simulink model "AllCheckoutsSim"  (R2020a)
settings: Solver=VariableStepAuto  StartTime=0.0  StopTime=2000000  RelTol=1e-3
InitFcn:
  | SimulationParameters
values from neighbouring files (symbols this model uses):
  NumExpressCheckouts = 2    [Sandbox.m]    (also in SimWrapper.m = NumExpressCheckoutsVec(i); SimulationParameters.m = Inputs(2))
  NumExpressCheckoutsHelper = NumExpressCheckouts    (= 2)    [Sandbox.m]    (also in SimulationParameters.m = NumExpressCheckouts)
  NumRegularCheckouts = 7    [Sandbox.m]    (also in SimWrapper.m = NumRegularCheckoutsVec(i); SimulationParameters.m = Inputs(1))
  NumRegularCheckoutsHelper = NumRegularCheckouts    (= 7)    [Sandbox.m]    (also in SimulationParameters.m = NumRegularCheckouts)
  NumSelfCheckouts = 2    [Sandbox.m]    (also in SimWrapper.m = NumSelfCheckoutsVec(i); SimulationParameters.m = Inputs(3))
  NumSelfCheckoutsHelper = NumSelfCheckouts    (= 2)    [Sandbox.m]    (also in SimulationParameters.m = NumSelfCheckouts)
  QueueCapacity = 7    [Sandbox.m]    (also in SimWrapper.m = QueueCapacityVec(i); SimulationParameters.m = Inputs(4))
undefined symbols (not defined in the file or in its folder): m, n
libraries: dspindex x3, dspstat3 x3
settings Model: Creator=jggam  LastModifiedBy=jggam

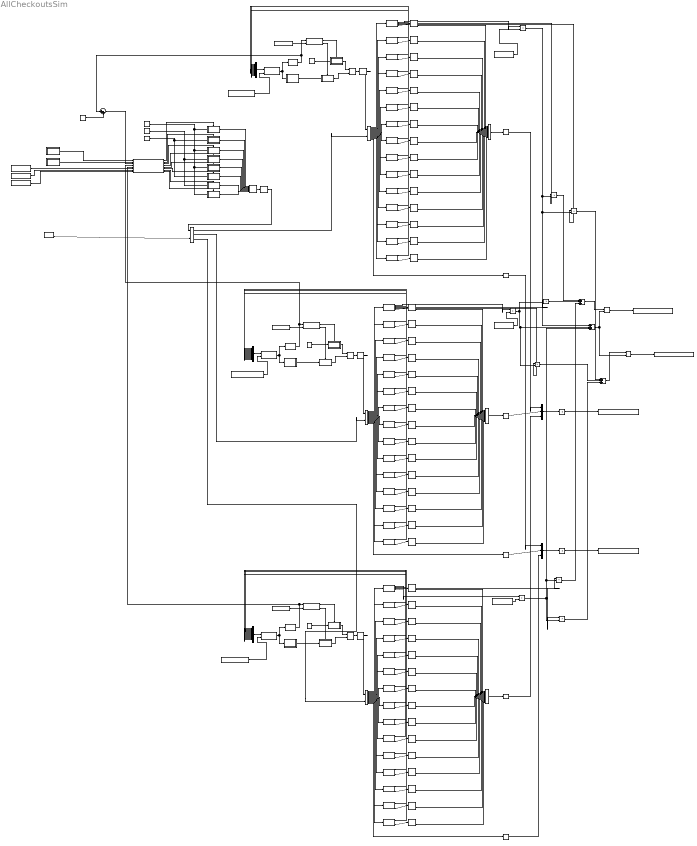
== system AllCheckoutsSim ==
  note: u1 = BelowItemsThresh
      | u2 = SelfCheckoutEligibile
      | u3 = Min Length of Regular
      | u4 = Min Length of Express
      | u5 = Min Length of Self
      | u6 = NumRegularCheckouts
      | u7 = NumExpressCheckouts
      | u8 = NumSelfCheckouts
  note: Hello! Welcome to the simulation of checkouts at a grocery store.
      | In order to change the queue capacities, number of each type of checkouts, item limit, and time of day,
      | 	change the variables at the top of the SimulationParameters.m file in MATLAB.
      |
      | You can have between 0 and 15 checkouts of each type, but make sure to always use at least 1 regular checkout.
      | Generally, your wait times will get much shorter is you use more than 9 or 10 total checkouts.
      |
      | You don't need to run the file, just change the variables and save the file.
      | After saving the SimulationParameters.m file, you can open the Data Inspector at the top of Simulink,
      | 	then Run the simulation.
      |
      | In the Data Inspector, there are a few signals that you can view. If you sort the signals by Name, they'll be grouped by type.
      | 	A. Average wait times for each type of checkout and overall.
      | 	B. Number of customers serviced by each type of checkout and overall.
      | 	C. Number of customers lost by each type of checkout and overall. I would only use the overall value here.
      | 	D. Average number of customers for each type of checkout and overall.
      | 	E. Current number of customers over time for each type of checkout and overall.
      | 	F. Total customers arrived to the simulation.
  A. Overall Average Wait Time : Product  Inputs=*/
  Add : Sum  Inputs=+++
  Add1 : Sum  Inputs=+++
  Add2 : Sum  Inputs=+++
  Aggregate all queue lengths : Concatenate  NumInputs=15
  Aggregate all queue lengths1 : Concatenate  NumInputs=15
  Aggregate all queue lengths2 : Concatenate  NumInputs=15
  B. Express Serviced Customers : EntityTerminator  InputPortMessageModes=m  NumberEntitiesArrived=on
      settings: OutputPortMap=o0
  B. Regular Serviced Customers : EntityTerminator  InputPortMessageModes=m  NumberEntitiesArrived=on
      settings: OutputPortMap=o0
  B. Self Serviced Customers : EntityTerminator  InputPortMessageModes=m  NumberEntitiesArrived=on
      settings: OutputPortMap=o0
  B. Total Serviced Customers : Sum  Inputs=+
  C. Express Lost Customers : EntityTerminator  InputPortMessageModes=m  NumberEntitiesArrived=on
      settings: OutputPortMap=o0
  C. Regular Lost Customers : EntityTerminator  InputPortMessageModes=m  NumberEntitiesArrived=on
      settings: OutputPortMap=o0
  C. Self Lost Customers : EntityTerminator  InputPortMessageModes=m  NumberEntitiesArrived=on
      settings: OutputPortMap=o0
  C. Total Lost Customers : Sum  Inputs=+
  Concatenate : Concatenate  NumInputs=3
  Concatenate1 : Concatenate  NumInputs=3
  Constant : Constant  Value=QueueCapacity
  Constant1 : Constant  Value=QueueCapacity
  Constant10 : Constant  Value=[1:NumSelfCheckoutsHelper]
  Constant13 : Constant  Value=[1:NumExpressCheckoutsHelper]
  Constant2 : Constant  Value=QueueCapacity
  Constant3 : Constant  Value=NumRegularCheckouts
  Constant4 : Constant  Value=NumRegularCheckouts
  Constant5 : Constant  Value=NumExpressCheckouts
  Constant6 : Constant  Value=NumExpressCheckouts
  Constant7 : Constant  Value=NumSelfCheckouts
  Constant8 : Constant  Value=[1:NumRegularCheckoutsHelper]
  Constant9 : Constant  Value=NumSelfCheckouts
  Customer Arrivals : EntityGenerator  OutputPortMessageModes=n,m  TimeSource=MATLAB action  Period=0.5  IntergenerationTimeAction=dt = arrivalTime(RandArrivalTimesDist);  GenerateEntityAtSimulationStart=off  GenerateAction=|  ExitAction=|  AttributeName=NumberOfItems|BelowItemThresh|SelfCheckoutEligible  AttributeInitialValue=1|false|false  NumberEntitiesDeparted=on  EntityType=Structured  EntityTypeName=Entity
      GenerateAction=|
      | entity.NumberOfItems = numberOfItems(RandItemsDist);
      | if entity.NumberOfItems <= SelfAndExpressMaxItems
      |     entity.BelowItemThresh = true;
      | end
      | if rand() < AmountSelfCheckoutEligible
      |     entity.SelfCheckoutEligible = true;
      | end
      ExitAction=|
      | observeBelowItemThresh(entity.BelowItemThresh);
      | observeEligibility(entity.SelfCheckoutEligible);
      settings: OutputPortMap=o0,o3
  D. Overall Average # of Customers Waiting : Product  Inputs=*/
  Determine which queue to send to : Merge
  Determine which queue to send to1 : Merge
  Determine which queue to send to2 : Merge
  Entity Input Switch : EntityInputSwitch  InputPortMessageModes=m,m,m,m,m,m,m,m,m,m,m,m,m,m,m  OutputPortMessageModes=m  NumberInputPorts=15
      settings: InputPortMap=u1,u2,u3,u4,u5,u6,u7,u8,u9,u10,u11,u12,u13,u14,u15
  Entity Input Switch1 : EntityInputSwitch  InputPortMessageModes=m,m,m,m,m,m,m,m,m,m,m,m,m,m,m  OutputPortMessageModes=m  NumberInputPorts=15
      settings: InputPortMap=u1,u2,u3,u4,u5,u6,u7,u8,u9,u10,u11,u12,u13,u14,u15
  Entity Input Switch2 : EntityInputSwitch  InputPortMessageModes=m,m,m,m,m,m,m,m,m,m,m,m,m,m,m  OutputPortMessageModes=m  NumberInputPorts=15
      settings: InputPortMap=u1,u2,u3,u4,u5,u6,u7,u8,u9,u10,u11,u12,u13,u14,u15
  Entity Output Switch : EntityOutputSwitch  InputPortMessageModes=m,m  OutputPortMessageModes=m,m,m,m,m,m,m,m,m,m,m,m,m,m,m,m  NumberOutputPorts=16  SwitchingCriterion=From control port  SwitchAttributeName=Attribute1
      settings: InputPortMap=u0,u1  OutputPortMap=o0,o1,o2,o3,o4,o5,o6,o7,o8,o9,o10,o11,o12,o13,o14,o15
  Entity Output Switch1 : EntityOutputSwitch  InputPortMessageModes=m,m  OutputPortMessageModes=m,m,m,m,m,m,m,m,m,m,m,m,m,m,m,m  NumberOutputPorts=16  SwitchingCriterion=From control port  SwitchAttributeName=Attribute1
      settings: InputPortMap=u0,u1  OutputPortMap=o0,o1,o2,o3,o4,o5,o6,o7,o8,o9,o10,o11,o12,o13,o14,o15
  Entity Output Switch2 : EntityOutputSwitch  InputPortMessageModes=m,m  OutputPortMessageModes=m,m,m,m,m,m,m,m,m,m,m,m,m,m,m,m  NumberOutputPorts=16  SwitchingCriterion=From control port  SwitchAttributeName=Attribute1
      settings: InputPortMap=u0,u1  OutputPortMap=o0,o1,o2,o3,o4,o5,o6,o7,o8,o9,o10,o11,o12,o13,o14,o15
  Entity Output Switch3 : EntityOutputSwitch  InputPortMessageModes=m,m  OutputPortMessageModes=m,m,m  NumberOutputPorts=3  SwitchingCriterion=From control port  SwitchAttributeName=Attribute1
      settings: InputPortMap=u0,u1  OutputPortMap=o0,o1,o2
  Express Checkout : Constant  Value=2
  Express Queue1 : Queue  InputPortMessageModes=m  OutputPortMessageModes=n,n,n,n,m  Capacity=QueueCapacity  NumberEntitiesDeparted=on  NumberEntitiesInBlock=on  AverageWait=on  AverageQueueLength=on
      settings: OutputPortMap=o0,o1,o2,o3,o5
  Express Queue{2..15} (14 alike) : Queue  InputPortMessageModes=m  OutputPortMessageModes=n,n,n,m  Capacity=QueueCapacity  NumberEntitiesInBlock=on  AverageWait=on  AverageQueueLength=on
      settings: OutputPortMap=o1,o2,o3,o5
  Express Server{1..15} (15 alike) : EntityServer  InputPortMessageModes=m  OutputPortMessageModes=n,m  Capacity=1  ServiceTimeSource=MATLAB action  ServiceTimeValue=1.75  ServiceTimeAction=dt = expressServiceTime(RandExpressServiceTimesDist);  AverageWait=on
      settings: OutputPortMap=o4,o9
  Go to Regular : Subsystem  TreatAsAtomicUnit=on
  If : If  NumInputs=2  IfExpression=u1 == u2  ZeroCross=off
  If for self checkouts : If  NumInputs=8  IfExpression=u7 == 0 & u8 == 0  ElseIfExpressions=u7 == 0 & u1 & u2 & u5 <= u3, u7 == 0, u8 == 0 & u1 & u4 <= u3, u8 == 0, u1 & u2 & u5 <= u3 & u5 <= u4, u1 & u4 <= u3  ZeroCross=off
  "If shortest queue is full, remove this customer" : Subsystem  TreatAsAtomicUnit=on
  "If shortest queue is full, remove this customer1" : Subsystem  TreatAsAtomicUnit=on
  "If shortest queue is full, remove this customer2" : Subsystem  TreatAsAtomicUnit=on
  "If there are no express or self, send to regular" : Subsystem  TreatAsAtomicUnit=on
  "If there are no express, and we're under items limit, and we're eligible for self, and the regular queues aren't shorter than self, go to self" : Subsystem  TreatAsAtomicUnit=on
  "If there are no express, go to regular" : Subsystem  TreatAsAtomicUnit=on
  "If there are no self, and we're under the items limit, and the regular queues aren't shorter than express, go to express" : Subsystem  TreatAsAtomicUnit=on
  "If there are no self, go to regular" : Subsystem  TreatAsAtomicUnit=on
  "If we're under the items limit and eligible for self and the regular and express queues aren't shorter than self, go to self" : Subsystem  TreatAsAtomicUnit=on
  "If we're under the items limit and the regular queue isn't shorter than express, go to express" : Subsystem  TreatAsAtomicUnit=on
  If1 : If  NumInputs=2  IfExpression=u1 == u2  ZeroCross=off
  If2 : If  NumInputs=2  IfExpression=u1 == u2  ZeroCross=off
  Index of exit queue : Constant  Value=16
  Index of exit queue1 : Constant  Value=16
  Index of exit queue2 : Constant  Value=16
  Only use open registers : dspindex/Variable Selector  NumInputs=1  rowsOrCols=Rows  IdxMode=Variable  Elements=16  ZerOneIdxMode=One-based  errmode=Clip Index  FillMode=off  FillValues=0
  Only use open registers1 : dspindex/Variable Selector  NumInputs=1  rowsOrCols=Rows  IdxMode=Variable  Elements=[16]  ZerOneIdxMode=One-based  errmode=Clip Index  FillMode=on  FillValues=0
  Only use open registers2 : dspindex/Variable Selector  NumInputs=1  rowsOrCols=Rows  IdxMode=Variable  Elements=[16]  ZerOneIdxMode=One-based  errmode=Clip Index  FillMode=on  FillValues=0
  "Otherwise, send customer to random shortest queue" : Subsystem  TreatAsAtomicUnit=on
  "Otherwise, send customer to random shortest queue1" : Subsystem  TreatAsAtomicUnit=on
  "Otherwise, send customer to random shortest queue2" : Subsystem  TreatAsAtomicUnit=on
  Product{,1..8} (9 alike) : Product
  Random index of shortest queue length : MATLAB Function  TreatAsAtomicUnit=on
  Random index of shortest queue length1 : MATLAB Function  TreatAsAtomicUnit=on
  Random index of shortest queue length2 : MATLAB Function  TreatAsAtomicUnit=on
  Regular Checkout : Constant
  Regular Checkout Offset : Constant  Value=0
  Regular Queue1 : Queue  InputPortMessageModes=m  OutputPortMessageModes=n,n,n,n,m  Capacity=QueueCapacity  NumberEntitiesDeparted=on  NumberEntitiesInBlock=on  AverageWait=on  AverageQueueLength=on
      settings: OutputPortMap=o0,o1,o2,o3,o5
  Regular Queue{2..15} (14 alike) : Queue  InputPortMessageModes=m  OutputPortMessageModes=n,n,n,m  Capacity=QueueCapacity  NumberEntitiesInBlock=on  AverageWait=on  AverageQueueLength=on
      settings: OutputPortMap=o1,o2,o3,o5
  Regular Server1 : EntityServer  InputPortMessageModes=m  OutputPortMessageModes=n,m  Capacity=1  ServiceTimeSource=MATLAB action  ServiceTimeValue=1.75  ServiceTimeAction=|  AverageWait=on
      | if entity.BelowItemThresh
      |     dt = expressServiceTime(RandExpressServiceTimesDist);
      | else
      |     dt = regularServiceTime(RandRegularServiceTimesDist);
      settings: OutputPortMap=o4,o9
  Regular Server10 : EntityServer  InputPortMessageModes=m  OutputPortMessageModes=n,m  Capacity=1  ServiceTimeSource=MATLAB action  ServiceTimeValue=1.75  ServiceTimeAction=|  AverageWait=on
      | if entity.BelowItemThresh
      |     dt = expressServiceTime(RandExpressServiceTimesDist);
      | else
      |     dt = regularServiceTime(RandRegularServiceTimesDist);
      settings: OutputPortMap=o4,o9
  Regular Server11 : EntityServer  InputPortMessageModes=m  OutputPortMessageModes=n,m  Capacity=1  ServiceTimeSource=MATLAB action  ServiceTimeValue=1.75  ServiceTimeAction=|  AverageWait=on
      | if entity.BelowItemThresh
      |     dt = expressServiceTime(RandExpressServiceTimesDist);
      | else
      |     dt = regularServiceTime(RandRegularServiceTimesDist);
      settings: OutputPortMap=o4,o9
  Regular Server12 : EntityServer  InputPortMessageModes=m  OutputPortMessageModes=n,m  Capacity=1  ServiceTimeSource=MATLAB action  ServiceTimeValue=1.75  ServiceTimeAction=|  AverageWait=on
      | if entity.BelowItemThresh
      |     dt = expressServiceTime(RandExpressServiceTimesDist);
      | else
      |     dt = regularServiceTime(RandRegularServiceTimesDist);
      settings: OutputPortMap=o4,o9
  Regular Server13 : EntityServer  InputPortMessageModes=m  OutputPortMessageModes=n,m  Capacity=1  ServiceTimeSource=MATLAB action  ServiceTimeValue=1.75  ServiceTimeAction=|  AverageWait=on
      | if entity.BelowItemThresh
      |     dt = expressServiceTime(RandExpressServiceTimesDist);
      | else
      |     dt = regularServiceTime(RandRegularServiceTimesDist);
      settings: OutputPortMap=o4,o9
  Regular Server14 : EntityServer  InputPortMessageModes=m  OutputPortMessageModes=n,m  Capacity=1  ServiceTimeSource=MATLAB action  ServiceTimeValue=1.75  ServiceTimeAction=|  AverageWait=on
      | if entity.BelowItemThresh
      |     dt = expressServiceTime(RandExpressServiceTimesDist);
      | else
      |     dt = regularServiceTime(RandRegularServiceTimesDist);
      settings: OutputPortMap=o4,o9
  Regular Server15 : EntityServer  InputPortMessageModes=m  OutputPortMessageModes=n,m  Capacity=1  ServiceTimeSource=MATLAB action  ServiceTimeValue=1.75  ServiceTimeAction=|  AverageWait=on
      | if entity.BelowItemThresh
      |     dt = expressServiceTime(RandExpressServiceTimesDist);
      | else
      |     dt = regularServiceTime(RandRegularServiceTimesDist);
      settings: OutputPortMap=o4,o9
  Regular Server2 : EntityServer  InputPortMessageModes=m  OutputPortMessageModes=n,m  Capacity=1  ServiceTimeSource=MATLAB action  ServiceTimeValue=1.75  ServiceTimeAction=|  AverageWait=on
      | if entity.BelowItemThresh
      |     dt = expressServiceTime(RandExpressServiceTimesDist);
      | else
      |     dt = regularServiceTime(RandRegularServiceTimesDist);
      settings: OutputPortMap=o4,o9
  Regular Server3 : EntityServer  InputPortMessageModes=m  OutputPortMessageModes=n,m  Capacity=1  ServiceTimeSource=MATLAB action  ServiceTimeValue=1.75  ServiceTimeAction=|  AverageWait=on
      | if entity.BelowItemThresh
      |     dt = expressServiceTime(RandExpressServiceTimesDist);
      | else
      |     dt = regularServiceTime(RandRegularServiceTimesDist);
      settings: OutputPortMap=o4,o9
  Regular Server4 : EntityServer  InputPortMessageModes=m  OutputPortMessageModes=n,m  Capacity=1  ServiceTimeSource=MATLAB action  ServiceTimeValue=1.75  ServiceTimeAction=|  AverageWait=on
      | if entity.BelowItemThresh
      |     dt = expressServiceTime(RandExpressServiceTimesDist);
      | else
      |     dt = regularServiceTime(RandRegularServiceTimesDist);
      settings: OutputPortMap=o4,o9
  Regular Server5 : EntityServer  InputPortMessageModes=m  OutputPortMessageModes=n,m  Capacity=1  ServiceTimeSource=MATLAB action  ServiceTimeValue=1.75  ServiceTimeAction=|  AverageWait=on
      | if entity.BelowItemThresh
      |     dt = expressServiceTime(RandExpressServiceTimesDist);
      | else
      |     dt = regularServiceTime(RandRegularServiceTimesDist);
      settings: OutputPortMap=o4,o9
  Regular Server6 : EntityServer  InputPortMessageModes=m  OutputPortMessageModes=n,m  Capacity=1  ServiceTimeSource=MATLAB action  ServiceTimeValue=1.75  ServiceTimeAction=|  AverageWait=on
      | if entity.BelowItemThresh
      |     dt = expressServiceTime(RandExpressServiceTimesDist);
      | else
      |     dt = regularServiceTime(RandRegularServiceTimesDist);
      settings: OutputPortMap=o4,o9
  Regular Server7 : EntityServer  InputPortMessageModes=m  OutputPortMessageModes=n,m  Capacity=1  ServiceTimeSource=MATLAB action  ServiceTimeValue=1.75  ServiceTimeAction=|  AverageWait=on
      | if entity.BelowItemThresh
      |     dt = expressServiceTime(RandExpressServiceTimesDist);
      | else
      |     dt = regularServiceTime(RandRegularServiceTimesDist);
      settings: OutputPortMap=o4,o9
  Regular Server8 : EntityServer  InputPortMessageModes=m  OutputPortMessageModes=n,m  Capacity=1  ServiceTimeSource=MATLAB action  ServiceTimeValue=1.75  ServiceTimeAction=|  AverageWait=on
      | if entity.BelowItemThresh
      |     dt = expressServiceTime(RandExpressServiceTimesDist);
      | else
      |     dt = regularServiceTime(RandRegularServiceTimesDist);
      settings: OutputPortMap=o4,o9
  Regular Server9 : EntityServer  InputPortMessageModes=m  OutputPortMessageModes=n,m  Capacity=1  ServiceTimeSource=MATLAB action  ServiceTimeValue=1.75  ServiceTimeAction=|  AverageWait=on
      | if entity.BelowItemThresh
      |     dt = expressServiceTime(RandExpressServiceTimesDist);
      | else
      |     dt = regularServiceTime(RandRegularServiceTimesDist);
      settings: OutputPortMap=o4,o9
  Self Checkout : Constant  Value=3
  Self Queue1 : Queue  InputPortMessageModes=m  OutputPortMessageModes=n,n,n,n,m  Capacity=QueueCapacity  NumberEntitiesDeparted=on  NumberEntitiesInBlock=on  AverageWait=on  AverageQueueLength=on
      settings: OutputPortMap=o0,o1,o2,o3,o5
  Self Queue{2..15} (14 alike) : Queue  InputPortMessageModes=m  OutputPortMessageModes=n,n,n,m  Capacity=QueueCapacity  NumberEntitiesInBlock=on  AverageWait=on  AverageQueueLength=on
      settings: OutputPortMap=o1,o2,o3,o5
  Self Server{1..15} (15 alike) : EntityServer  InputPortMessageModes=m  OutputPortMessageModes=n,m  Capacity=1  ServiceTimeSource=MATLAB action  ServiceTimeValue=1.75  ServiceTimeAction=dt = selfServiceTime(RandSelfServiceTimesDist);  AverageWait=on
      settings: OutputPortMap=o4,o9
  Send{,1..3} (4 alike) : Send  OutputPortMessageModes=m
  Shortest Queue Length : dspstat3/Minimum  operation=minimum  fcn=Value  indexBase=One  operateOver=Entire input  Dimension=1  InputProcessing=Columns as channels (frame based)  reset=None  roiEnable=off  roiType=Rectangles  roiPortion=Entire ROI  roiOutput=Individual statistics for each ROI  roiFlag=off  roundingMode=Floor  overflowMode=off
      settings: SourceProductBaseCode=DS
  Shortest Queue Length1 : dspstat3/Minimum  operation=minimum  fcn=Value  indexBase=One  operateOver=Entire input  Dimension=1  InputProcessing=Columns as channels (frame based)  reset=None  roiEnable=off  roiType=Rectangles  roiPortion=Entire ROI  roiOutput=Individual statistics for each ROI  roiFlag=off  roundingMode=Floor  overflowMode=off
      settings: SourceProductBaseCode=DS
  Shortest Queue Length2 : dspstat3/Minimum  operation=minimum  fcn=Value  indexBase=One  operateOver=Entire input  Dimension=1  InputProcessing=Columns as channels (frame based)  reset=None  roiEnable=off  roiType=Rectangles  roiPortion=Entire ROI  roiOutput=Individual statistics for each ROI  roiFlag=off  roundingMode=Floor  overflowMode=off
      settings: SourceProductBaseCode=DS
  Simulink Function : Subsystem  TreatAsAtomicUnit=on
  Simulink Function1 : Subsystem  TreatAsAtomicUnit=on
  Sum : Sum  Inputs=|++
  To Workspace : ToWorkspace  VariableName=OverallAverageWaitTime  SaveFormat=Timeseries  SampleTime=-1
      settings: MaxDataPoints=1
  To Workspace1 : ToWorkspace  VariableName=OverallAverageNumCustomersWaiting  SaveFormat=Timeseries  SampleTime=-1
      settings: MaxDataPoints=1
  To Workspace2 : ToWorkspace  VariableName=OverallNumCustomersServiced  SaveFormat=Timeseries  SampleTime=-1
      settings: MaxDataPoints=1
  To Workspace3 : ToWorkspace  VariableName=OverallNumCustomersLost  SaveFormat=Timeseries  SampleTime=-1
      settings: MaxDataPoints=1
  merge1 : Merge  Inputs=8
  wires:
  Regular Queue1/5 -> Regular Server1/1
  Entity Input Switch/1 -> B. Regular Serviced Customers/1
  Send/1 -> Entity Output Switch/1
  Regular Queue1/2 -> Aggregate all queue lengths/1
  Regular Queue2/4 -> Regular Server2/1
  Regular Queue3/4 -> Regular Server3/1
  Regular Queue4/4 -> Regular Server4/1
  Regular Queue5/4 -> Regular Server5/1
  Regular Queue6/4 -> Regular Server6/1
  Regular Queue7/4 -> Regular Server7/1
  Regular Queue8/4 -> Regular Server8/1
  Regular Queue9/4 -> Regular Server9/1
  Regular Queue10/4 -> Regular Server10/1
  Regular Queue11/4 -> Regular Server11/1
  Regular Queue12/4 -> Regular Server12/1
  Regular Queue13/4 -> Regular Server13/1
  Regular Queue14/4 -> Regular Server14/1
  Regular Queue15/4 -> Regular Server15/1
  Regular Server2/2 -> Entity Input Switch/2
  Regular Server3/2 -> Entity Input Switch/3
  Regular Server4/2 -> Entity Input Switch/4
  Regular Server5/2 -> Entity Input Switch/5
  Regular Server6/2 -> Entity Input Switch/6
  Regular Server7/2 -> Entity Input Switch/7
  Regular Server8/2 -> Entity Input Switch/8
  Regular Server9/2 -> Entity Input Switch/9
  Regular Server10/2 -> Entity Input Switch/10
  Regular Server11/2 -> Entity Input Switch/11
  Regular Server12/2 -> Entity Input Switch/12
  Regular Server13/2 -> Entity Input Switch/13
  Regular Server14/2 -> Entity Input Switch/14
  Regular Server15/2 -> Entity Input Switch/15
  Regular Queue2/1 -> Aggregate all queue lengths/2
  Regular Queue3/1 -> Aggregate all queue lengths/3
  Regular Queue4/1 -> Aggregate all queue lengths/4
  Regular Queue5/1 -> Aggregate all queue lengths/5
  Regular Queue6/1 -> Aggregate all queue lengths/6
  Regular Queue7/1 -> Aggregate all queue lengths/7
  Regular Queue8/1 -> Aggregate all queue lengths/8
  Regular Queue9/1 -> Aggregate all queue lengths/9
  Entity Output Switch/1 -> Regular Queue1/1
  Entity Output Switch/2 -> Regular Queue2/1
  Entity Output Switch/3 -> Regular Queue3/1
  Entity Output Switch/4 -> Regular Queue4/1
  Entity Output Switch/5 -> Regular Queue5/1
  Entity Output Switch/6 -> Regular Queue6/1
  Entity Output Switch/7 -> Regular Queue7/1
  Entity Output Switch/8 -> Regular Queue8/1
  Entity Output Switch/9 -> Regular Queue9/1
  Entity Output Switch/10 -> Regular Queue10/1
  Entity Output Switch/11 -> Regular Queue11/1
  Entity Output Switch/12 -> Regular Queue12/1
  Entity Output Switch/13 -> Regular Queue13/1
  Entity Output Switch/14 -> Regular Queue14/1
  Entity Output Switch/15 -> Regular Queue15/1
  Entity Output Switch/16 -> C. Regular Lost Customers/1
  Shortest Queue Length/1 -> Sum/1, If/1
  If/1 -> "If shortest queue is full, remove this customer"/Action
  If/2 -> "Otherwise, send customer to random shortest queue"/Action
  Regular Server1/2 -> Entity Input Switch/1
  Determine which queue to send to/1 -> Send/1
  Index of exit queue/1 -> "If shortest queue is full, remove this customer"/1(In1)
  "If shortest queue is full, remove this customer"/1(Out1) -> Determine which queue to send to/1
  Random index of shortest queue length/1(y) -> "Otherwise, send customer to random shortest queue"/1(In1)
  Regular Queue10/1 -> Aggregate all queue lengths/10
  Regular Queue11/1 -> Aggregate all queue lengths/11
  Regular Queue12/1 -> Aggregate all queue lengths/12
  Regular Queue13/1 -> Aggregate all queue lengths/13
  Regular Queue14/1 -> Aggregate all queue lengths/14
  Regular Queue15/1 -> Aggregate all queue lengths/15
  "Otherwise, send customer to random shortest queue"/1(Out1) -> Determine which queue to send to/2
  Constant/1 -> If/2
  Aggregate all queue lengths/1 -> Only use open registers/1
  Only use open registers/1 -> Random index of shortest queue length/1(u), Shortest Queue Length/1
  Shortest Queue Length1/1 -> If for self checkouts/4, If1/1
  Determine which queue to send to1/1 -> Send1/1
  Express Server10/2 -> Entity Input Switch1/10
  Express Server8/2 -> Entity Input Switch1/8
  Entity Output Switch1/6 -> Express Queue6/1
  Entity Output Switch1/8 -> Express Queue8/1
  Only use open registers1/1 -> Random index of shortest queue length1/1(u), Shortest Queue Length1/1
  Express Queue15/1 -> Aggregate all queue lengths1/15
  Aggregate all queue lengths1/1 -> Only use open registers1/1
  Express Queue13/1 -> Aggregate all queue lengths1/13
  Entity Output Switch1/5 -> Express Queue5/1
  Express Queue8/1 -> Aggregate all queue lengths1/8
  Express Server12/2 -> Entity Input Switch1/12
  Entity Output Switch1/15 -> Express Queue15/1
  Express Queue8/4 -> Express Server8/1
  Express Queue11/1 -> Aggregate all queue lengths1/11
  Express Queue14/4 -> Express Server14/1
  Express Queue14/1 -> Aggregate all queue lengths1/14
  Express Server2/2 -> Entity Input Switch1/2
  Entity Output Switch1/10 -> Express Queue10/1
  Express Queue11/4 -> Express Server11/1
  Random index of shortest queue length1/1(y) -> "Otherwise, send customer to random shortest queue1"/1(In1)
  Entity Output Switch1/16 -> C. Express Lost Customers/1
  Entity Output Switch1/3 -> Express Queue3/1
  Entity Output Switch1/7 -> Express Queue7/1
  Entity Output Switch1/12 -> Express Queue12/1
  Entity Output Switch1/4 -> Express Queue4/1
  Entity Output Switch1/14 -> Express Queue14/1
  Express Server9/2 -> Entity Input Switch1/9
  If1/2 -> "Otherwise, send customer to random shortest queue1"/Action
  Entity Output Switch1/11 -> Express Queue11/1
  Express Queue15/4 -> Express Server15/1
  Express Queue7/1 -> Aggregate all queue lengths1/7
  Entity Output Switch1/13 -> Express Queue13/1
  If1/1 -> "If shortest queue is full, remove this customer1"/Action
  Express Server6/2 -> Entity Input Switch1/6
  Express Server5/2 -> Entity Input Switch1/5
  Express Queue2/1 -> Aggregate all queue lengths1/2
  Express Queue6/1 -> Aggregate all queue lengths1/6
  Express Queue10/1 -> Aggregate all queue lengths1/10
  Express Server14/2 -> Entity Input Switch1/14
  "If shortest queue is full, remove this customer1"/1(Out1) -> Determine which queue to send to1/1
  Entity Output Switch1/2 -> Express Queue2/1
  Express Server15/2 -> Entity Input Switch1/15
  Index of exit queue1/1 -> "If shortest queue is full, remove this customer1"/1(In1)
  Express Server7/2 -> Entity Input Switch1/7
  Express Server13/2 -> Entity Input Switch1/13
  Express Server11/2 -> Entity Input Switch1/11
  Express Server4/2 -> Entity Input Switch1/4
  Express Queue13/4 -> Express Server13/1
  Express Queue3/1 -> Aggregate all queue lengths1/3
  Express Server3/2 -> Entity Input Switch1/3
  Express Queue4/4 -> Express Server4/1
  Express Queue9/1 -> Aggregate all queue lengths1/9
  Express Server1/2 -> Entity Input Switch1/1
  Express Queue4/1 -> Aggregate all queue lengths1/4
  Express Queue2/4 -> Express Server2/1
  "Otherwise, send customer to random shortest queue1"/1(Out1) -> Determine which queue to send to1/2
  Express Queue1/2 -> Aggregate all queue lengths1/1
  Express Queue9/4 -> Express Server9/1
  Send1/1 -> Entity Output Switch1/1
  Entity Output Switch1/1 -> Express Queue1/1
  Express Queue5/4 -> Express Server5/1
  Constant1/1 -> If1/2
  Express Queue6/4 -> Express Server6/1
  Express Queue10/4 -> Express Server10/1
  Express Queue5/1 -> Aggregate all queue lengths1/5
  Express Queue7/4 -> Express Server7/1
  Express Queue1/5 -> Express Server1/1
  Express Queue12/4 -> Express Server12/1
  Express Queue12/1 -> Aggregate all queue lengths1/12
  Express Queue3/4 -> Express Server3/1
  Entity Output Switch1/9 -> Express Queue9/1
  Entity Input Switch1/1 -> B. Express Serviced Customers/1
  Self Queue5/1 -> Aggregate all queue lengths2/5
  Self Queue13/4 -> Self Server13/1
  Self Queue13/1 -> Aggregate all queue lengths2/13
  Entity Output Switch2/13 -> Self Queue13/1
  Self Queue12/4 -> Self Server12/1
  Self Queue9/1 -> Aggregate all queue lengths2/9
  Self Queue9/4 -> Self Server9/1
  Entity Output Switch2/9 -> Self Queue9/1
  Entity Output Switch2/12 -> Self Queue12/1
  Self Server12/2 -> Entity Input Switch2/12
  Self Server7/2 -> Entity Input Switch2/7
  Entity Output Switch2/11 -> Self Queue11/1
  Self Queue11/1 -> Aggregate all queue lengths2/11
  Entity Output Switch2/2 -> Self Queue2/1
  Entity Output Switch2/10 -> Self Queue10/1
  Entity Output Switch2/14 -> Self Queue14/1
  Self Queue14/4 -> Self Server14/1
  Self Queue14/1 -> Aggregate all queue lengths2/14
  Self Queue6/1 -> Aggregate all queue lengths2/6
  Self Queue8/1 -> Aggregate all queue lengths2/8
  Self Queue5/4 -> Self Server5/1
  Entity Output Switch2/4 -> Self Queue4/1
  Self Queue3/4 -> Self Server3/1
  Entity Output Switch2/3 -> Self Queue3/1
  Self Queue3/1 -> Aggregate all queue lengths2/3
  Self Server3/2 -> Entity Input Switch2/3
  Self Server14/2 -> Entity Input Switch2/14
  Entity Output Switch2/7 -> Self Queue7/1
  Self Queue8/4 -> Self Server8/1
  Self Server13/2 -> Entity Input Switch2/13
  Entity Output Switch2/5 -> Self Queue5/1
  Self Server8/2 -> Entity Input Switch2/8
  Self Server4/2 -> Entity Input Switch2/4
  Self Server6/2 -> Entity Input Switch2/6
  Self Queue2/1 -> Aggregate all queue lengths2/2
  Entity Output Switch2/6 -> Self Queue6/1
  Self Server2/2 -> Entity Input Switch2/2
  Entity Input Switch2/1 -> B. Self Serviced Customers/1
  Self Queue7/4 -> Self Server7/1
  "Otherwise, send customer to random shortest queue2"/1(Out1) -> Determine which queue to send to2/2
  Entity Output Switch2/1 -> Self Queue1/1
  Self Queue1/2 -> Aggregate all queue lengths2/1
  Self Server11/2 -> Entity Input Switch2/11
  Self Server9/2 -> Entity Input Switch2/9
  Constant2/1 -> If2/2
  Self Server1/2 -> Entity Input Switch2/1
  Index of exit queue2/1 -> "If shortest queue is full, remove this customer2"/1(In1)
  "If shortest queue is full, remove this customer2"/1(Out1) -> Determine which queue to send to2/1
  If2/1 -> "If shortest queue is full, remove this customer2"/Action
  If2/2 -> "Otherwise, send customer to random shortest queue2"/Action
  Entity Output Switch2/8 -> Self Queue8/1
  Self Queue11/4 -> Self Server11/1
  Self Queue15/4 -> Self Server15/1
  Random index of shortest queue length2/1(y) -> "Otherwise, send customer to random shortest queue2"/1(In1)
  Self Queue7/1 -> Aggregate all queue lengths2/7
  Entity Output Switch2/16 -> C. Self Lost Customers/1
  Self Queue4/4 -> Self Server4/1
  Entity Output Switch2/15 -> Self Queue15/1
  Send2/1 -> Entity Output Switch2/1
  Self Queue6/4 -> Self Server6/1
  Determine which queue to send to2/1 -> Send2/1
  Self Server15/2 -> Entity Input Switch2/15
  Only use open registers2/1 -> Random index of shortest queue length2/1(u), Shortest Queue Length2/1
  Self Queue2/4 -> Self Server2/1
  Aggregate all queue lengths2/1 -> Only use open registers2/1
  Self Queue4/1 -> Aggregate all queue lengths2/4
  Self Queue10/1 -> Aggregate all queue lengths2/10
  Self Queue12/1 -> Aggregate all queue lengths2/12
  Self Queue10/4 -> Self Server10/1
  Self Queue15/1 -> Aggregate all queue lengths2/15
  Self Server5/2 -> Entity Input Switch2/5
  Self Server10/2 -> Entity Input Switch2/10
  Shortest Queue Length2/1 -> If for self checkouts/5, If2/1
  Self Queue1/5 -> Self Server1/1
  Entity Output Switch3/1 -> Entity Output Switch/2
  Entity Output Switch3/2 -> Entity Output Switch1/2
  Customer Arrivals/2 -> Entity Output Switch3/2
  Simulink Function/1(Out1) -> If for self checkouts/1
  Simulink Function1/1(Out1) -> If for self checkouts/2
  Constant3/1 -> If for self checkouts/6
  Constant6/1 -> If for self checkouts/7
  Constant7/1 -> If for self checkouts/8
  If for self checkouts/1 -> "If there are no express or self, send to regular"/Action
  If for self checkouts/2 -> "If there are no express, and we're under items limit, and we're eligible for self, and the regular queues aren't shorter than self, go to self"/Action
  If for self checkouts/4 -> "If there are no self, and we're under the items limit, and the regular queues aren't shorter than express, go to express"/Action
  If for self checkouts/7 -> "If we're under the items limit and the regular queue isn't shorter than express, go to express"/Action
  If for self checkouts/6 -> "If we're under the items limit and eligible for self and the regular and express queues aren't shorter than self, go to self"/Action
  If for self checkouts/8 -> Go to Regular/Action
  Entity Output Switch3/3 -> Entity Output Switch2/2
  merge1/1 -> Send3/1
  Send3/1 -> Entity Output Switch3/1
  If for self checkouts/3 -> "If there are no express, go to regular"/Action
  If for self checkouts/5 -> "If there are no self, go to regular"/Action
  Constant13/1 -> Only use open registers1/2
  Constant10/1 -> Only use open registers2/2
  Constant8/1 -> Only use open registers/2
  B. Regular Serviced Customers/1 -> Concatenate/1
  B. Express Serviced Customers/1 -> Concatenate/2
  B. Self Serviced Customers/1 -> Concatenate/3
  Concatenate/1 -> B. Total Serviced Customers/1
  C. Express Lost Customers/1 -> Concatenate1/2
  C. Self Lost Customers/1 -> Concatenate1/3
  Concatenate1/1 -> C. Total Lost Customers/1
  C. Regular Lost Customers/1 -> Concatenate1/1
  Regular Checkout Offset/1 -> Sum/2
  Sum/1 -> If for self checkouts/3
  Regular Queue1/3 -> Product/1
  Express Queue1/3 -> Product1/1
  Self Queue1/3 -> Product2/1
  Product/1 -> Add/1
  Product1/1 -> Add/2
  Product2/1 -> Add/3
  Add/1 -> A. Overall Average Wait Time/1
  Add1/1 -> D. Overall Average # of Customers Waiting/2, A. Overall Average Wait Time/2
  Regular Queue1/1 -> Product3/1
  Constant4/1 -> Product3/2
  Product3/1 -> Add1/1, Product6/2, Product/2
  Express Queue1/1 -> Product4/1
  Constant5/1 -> Product4/2
  Product4/1 -> Product7/2, Add1/2, Product1/2
  Self Queue1/1 -> Product5/1
  Constant9/1 -> Product5/2
  Product5/1 -> Product8/2, Add1/3, Product2/2
  "If there are no express or self, send to regular"/1(Out1) -> merge1/1
  "If there are no express, and we're under items limit, and we're eligible for self, and the regular queues aren't shorter than self, go to self"/1(Out1) -> merge1/2
  "If there are no express, go to regular"/1(Out1) -> merge1/3
  "If there are no self, and we're under the items limit, and the regular queues aren't shorter than express, go to express"/1(Out1) -> merge1/4
  "If there are no self, go to regular"/1(Out1) -> merge1/5
  "If we're under the items limit and eligible for self and the regular and express queues aren't shorter than self, go to self"/1(Out1) -> merge1/6
  "If we're under the items limit and the regular queue isn't shorter than express, go to express"/1(Out1) -> merge1/7
  Go to Regular/1(Out1) -> merge1/8
  Regular Checkout/1 -> Go to Regular/1(In1), "If there are no self, go to regular"/1(In1), "If there are no express, go to regular"/1(In1), "If there are no express or self, send to regular"/1(In1)
  Express Checkout/1 -> "If there are no self, and we're under the items limit, and the regular queues aren't shorter than express, go to express"/1(In1), "If we're under the items limit and the regular queue isn't shorter than express, go to express"/1(In1)
  Self Checkout/1 -> "If we're under the items limit and eligible for self and the regular and express queues aren't shorter than self, go to self"/1(In1), "If there are no express, and we're under items limit, and we're eligible for self, and the regular queues aren't shorter than self, go to self"/1(In1)
  Regular Queue1/4 -> Product6/1
  Express Queue1/4 -> Product7/1
  Self Queue1/4 -> Product8/1
  Product8/1 -> Add2/3
  Product7/1 -> Add2/2
  Product6/1 -> Add2/1
  Add2/1 -> D. Overall Average # of Customers Waiting/1
  A. Overall Average Wait Time/1 -> To Workspace/1
  D. Overall Average # of Customers Waiting/1 -> To Workspace1/1
  B. Total Serviced Customers/1 -> To Workspace2/1
  C. Total Lost Customers/1 -> To Workspace3/1

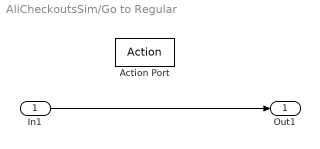
== system AllCheckoutsSim/Go to Regular ==
  In1 : Inport
  Action Port : ActionPort  ActionPortLabel=else
  Out1 : Outport
  wires:
  In1/1 -> Out1/1

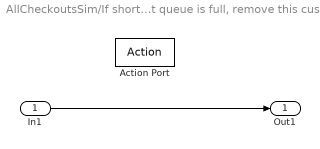
== system AllCheckoutsSim/If shortest queue is full, remove this customer ==
  In1 : Inport
  Action Port : ActionPort  ActionPortLabel=if(u1 == u2)
  Out1 : Outport
  wires:
  In1/1 -> Out1/1

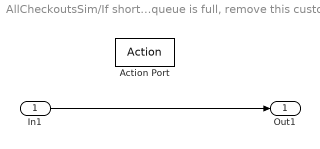
== system AllCheckoutsSim/If shortest queue is full, remove this customer1 ==
  In1 : Inport
  Action Port : ActionPort  ActionPortLabel=if(u1 == u2)
  Out1 : Outport
  wires:
  In1/1 -> Out1/1

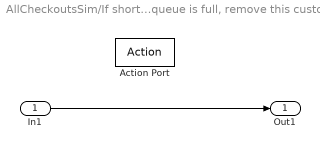
== system AllCheckoutsSim/If shortest queue is full, remove this customer2 ==
  In1 : Inport
  Action Port : ActionPort  ActionPortLabel=if(u1 == u2)
  Out1 : Outport
  wires:
  In1/1 -> Out1/1

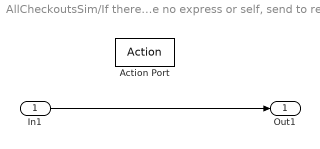
== system AllCheckoutsSim/If there are no express or self, send to regular ==
  In1 : Inport
  Action Port : ActionPort  ActionPortLabel=if(u7 == 0 & u8 == 0)
  Out1 : Outport
  wires:
  In1/1 -> Out1/1

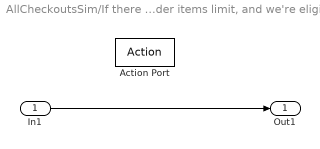
== system AllCheckoutsSim/If there are no express, and we're under items limit, and we're eligible for self, and the regular queues aren't shorter than self, go to self ==
  In1 : Inport
  Action Port : ActionPort  ActionPortLabel=elseif(u7 == 0 & u1 & u2 & u5 <= u3)
  Out1 : Outport
  wires:
  In1/1 -> Out1/1

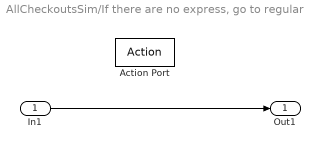
== system AllCheckoutsSim/If there are no express, go to regular ==
  In1 : Inport
  Action Port : ActionPort  ActionPortLabel=elseif( u7 == 0)
  Out1 : Outport
  wires:
  In1/1 -> Out1/1

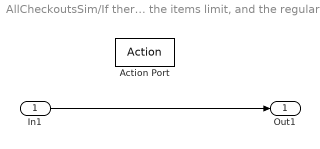
== system AllCheckoutsSim/If there are no self, and we're under the items limit, and the regular queues aren't shorter than express, go to express ==
  In1 : Inport
  Action Port : ActionPort  ActionPortLabel=elseif( u8 == 0 & u1 & u4 <= u3)
  Out1 : Outport
  wires:
  In1/1 -> Out1/1

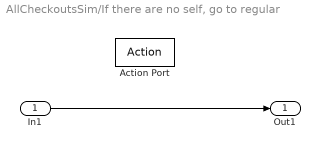
== system AllCheckoutsSim/If there are no self, go to regular ==
  In1 : Inport
  Action Port : ActionPort  ActionPortLabel=elseif( u8 == 0)
  Out1 : Outport
  wires:
  In1/1 -> Out1/1

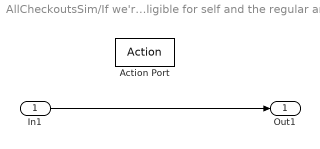
== system AllCheckoutsSim/If we're under the items limit and eligible for self and the regular and express queues aren't shorter than self, go to self ==
  In1 : Inport
  Action Port : ActionPort  ActionPortLabel=elseif( u1 & u2 & u5 <= u3 & u5 <= u4)
  Out1 : Outport
  wires:
  In1/1 -> Out1/1

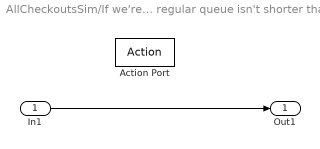
== system AllCheckoutsSim/If we're under the items limit and the regular queue isn't shorter than express, go to express ==
  In1 : Inport
  Action Port : ActionPort  ActionPortLabel=elseif( u1 & u4 <= u3)
  Out1 : Outport
  wires:
  In1/1 -> Out1/1

== system AllCheckoutsSim/Otherwise, send customer to random shortest queue ==
  In1 : Inport
  Action Port : ActionPort  ActionPortLabel=else
  Out1 : Outport
  wires:
  In1/1 -> Out1/1

== system AllCheckoutsSim/Otherwise, send customer to random shortest queue1 ==
  In1 : Inport
  Action Port : ActionPort  ActionPortLabel=else
  Out1 : Outport
  wires:
  In1/1 -> Out1/1

== system AllCheckoutsSim/Otherwise, send customer to random shortest queue2 ==
  In1 : Inport
  Action Port : ActionPort  ActionPortLabel=else
  Out1 : Outport
  wires:
  In1/1 -> Out1/1

== system AllCheckoutsSim/Simulink Function ==
  observeBelowItemThresh : TriggerPort  TriggerType=function-call  IsSimulinkFunction=on  FunctionName=observeBelowItemThresh  FunctionVisibility=scoped  VariantControl=(inherit)
  u : ArgIn  DisableCoverage=on  ArgumentName=u
  Out1 : Outport
  wires:
  u/1 -> Out1/1

== system AllCheckoutsSim/Simulink Function1 ==
  observeEligibility : TriggerPort  TriggerType=function-call  IsSimulinkFunction=on  FunctionName=observeEligibility  FunctionVisibility=scoped  VariantControl=(inherit)
  u : ArgIn  DisableCoverage=on  ArgumentName=u
  Out1 : Outport
  wires:
  u/1 -> Out1/1

== matlab function AllCheckoutsSim/Random index of shortest queue length ==
  data: u input; y output
function y = findAllMinLengthIndices(u)

indicies = find(u == min(u));
y = indicies(randi(length(indicies)));

== matlab function AllCheckoutsSim/Random index of shortest queue length2 ==
  data: u input; y output
function y = findAllMinLengthIndices(u)

indicies = find(u == min(u));
y = indicies(randi(length(indicies)));

== matlab function AllCheckoutsSim/Random index of shortest queue length1 ==
  data: u input; y output
function y = findAllMinLengthIndices(u)

indicies = find(u == min(u));
y = indicies(randi(length(indicies)));
